simulink model "SistemaCAS_v9"  (R2014a)
settings: Solver=ode3  StartTime=0.0  StopTime=100  RelTol=1e-3
settings Model: Creator=andre  LastModifiedBy=andre

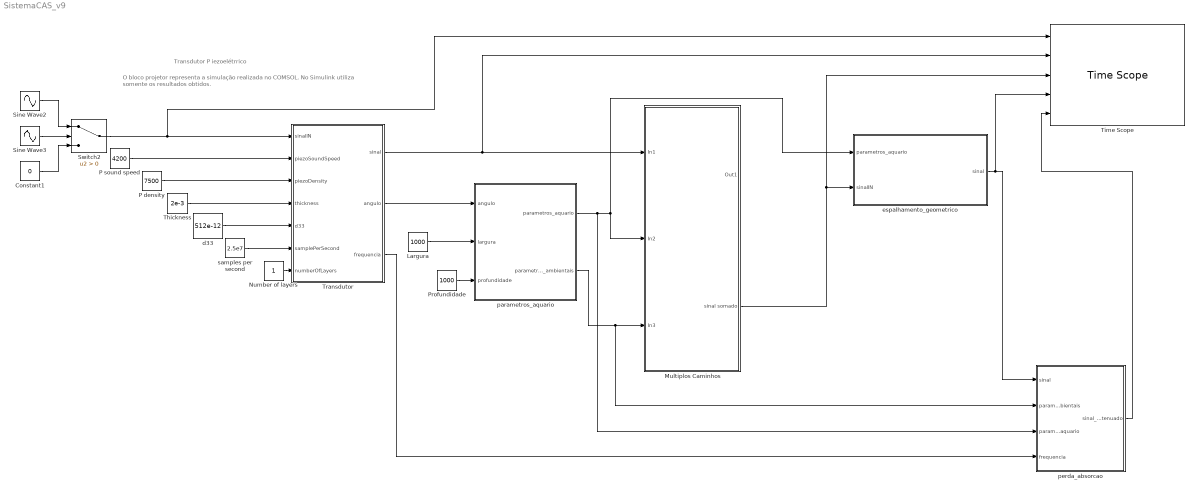
== system SistemaCAS_v9 ==
  note: O bloco projetor representa a simulação realizada no COMSOL. No Simulink utiliza somente os resultados obtidos.
  note: Transdutor P iezoelétrrico
  Constant1 : Constant  Value=0
  Largura : Constant  Value=1000
  Multiplos Caminhos : Subsystem
  Number of layers : Constant
  P density : Constant  Value=7500
  P sound speed : Constant  Value=4200
  Profundidade : Constant  Value=1000
  Sine Wave2 : Sin  SampleTime=0
  Sine Wave3 : Sin  SampleTime=0
  Switch2 : Switch  Criteria=u2 > Threshold
  Thickness : Constant  Value=2e-3
  Time Scope : TimeScope  NumInputPorts=5  DefaultConfigurationName=spbscopes.TimeScopeBlockCfg
  Transdutor : MATLAB Function  TreatAsAtomicUnit=on
  d33 : Constant  Value=512e-12
  espalhamento_geometrico : MATLAB Function  TreatAsAtomicUnit=on
  parametros_aquario : MATLAB Function  TreatAsAtomicUnit=on
  perda_absorcao : MATLAB Function  TreatAsAtomicUnit=on
  samples per second : Constant  Value=2.5e7
  wires:
  Largura/1 -> parametros_aquario/2(largura)
  Profundidade/1 -> parametros_aquario/3(profundidade)
  d33/1 -> Transdutor/5(d33)
  samples per second/1 -> Transdutor/6(samplePerSecond)
  Number of layers/1 -> Transdutor/7(numberOfLayers)
  P sound speed/1 -> Transdutor/2(piezoSoundSpeed)
  P density/1 -> Transdutor/3(piezoDensity)
  Thickness/1 -> Transdutor/4(thickness)
  Transdutor/2(angulo) -> parametros_aquario/1(angulo)
  Sine Wave2/1 -> Switch2/1
  Sine Wave3/1 -> Switch2/2
  Constant1/1 -> Switch2/3
  Switch2/1 -> Time Scope/1, Transdutor/1(sinalIN)
  Transdutor/1(sinal) -> Time Scope/2, Multiplos Caminhos/1(In1)
  parametros_aquario/1(parametros_aquario) -> perda_absorcao/3(parametros_aquario), Multiplos Caminhos/2(In2), espalhamento_geometrico/1(parametros_aquario)
  Multiplos Caminhos/2(sinal somado) -> Time Scope/3, espalhamento_geometrico/2(sinalIN)
  Transdutor/3(frequencia) -> perda_absorcao/4(frequencia)
  espalhamento_geometrico/1(sinal) -> Time Scope/4, perda_absorcao/1(sinal)
  parametros_aquario/2(parametros_ambientais) -> perda_absorcao/2(parametros_ambientais), Multiplos Caminhos/3(In3)
  perda_absorcao/1(sinal_atenuado) -> Time Scope/5

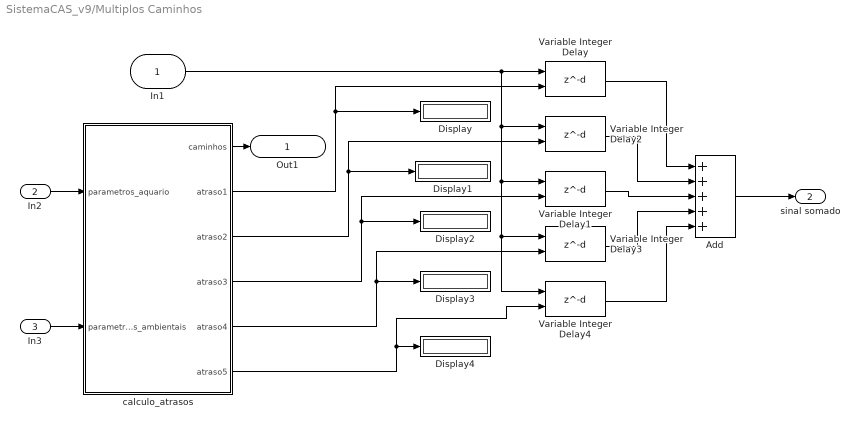
== system SistemaCAS_v9/Multiplos Caminhos ==
  In1 : Inport
  In2 : Inport  Port=2
  In3 : Inport  Port=3
  Add : Sum  Inputs=+++++
  Display{,1..4} (5 alike) : Display
  Variable Integer Delay{,1..4} (5 alike) : Delay  DelayLengthSource=Input port
      settings: InputPortMap=u0,p1
  calculo_atrasos : MATLAB Function  TreatAsAtomicUnit=on
  Out1 : Outport
  sinal somado : Outport  Port=2
  wires:
  calculo_atrasos/5(atraso4) -> Display3/1, Variable Integer Delay3/2
  calculo_atrasos/4(atraso3) -> Display2/1, Variable Integer Delay1/2
  In2/1 -> calculo_atrasos/1(parametros_aquario)
  In3/1 -> calculo_atrasos/2(parametros_ambientais)
  calculo_atrasos/1(caminhos) -> Out1/1
  In1/1 -> Variable Integer Delay4/1, Variable Integer Delay3/1, Variable Integer Delay1/1, Variable Integer Delay2/1, Variable Integer Delay/1
  calculo_atrasos/2(atraso1) -> Display/1, Variable Integer Delay/2
  calculo_atrasos/6(atraso5) -> Display4/1, Variable Integer Delay4/2
  Variable Integer Delay1/1 -> Add/3
  Variable Integer Delay2/1 -> Add/2
  Variable Integer Delay/1 -> Add/1
  Add/1 -> sinal somado/1
  calculo_atrasos/3(atraso2) -> Display1/1, Variable Integer Delay2/2
  Variable Integer Delay4/1 -> Add/5
  Variable Integer Delay3/1 -> Add/4

== matlab function SistemaCAS_v9/parametros_aquario ==
  data: angulo input; largura input; profundidade input; parametros_aquario output; parametros_ambientais output
function [parametros_aquario,parametros_ambientais] = parametros_aquario(angulo,largura,profundidade)
% consideraçoes para os parâmetros do aquário
% 1. emissor e receptor estão alinhados ( largura(x) e profundidade(z)
% iguais, só muda o comprimento (y)
% 2. o comprimento do aquario (L) é ideal para acontecer uma reflexão completa
% com o angulo de diretividade (que é o maior angulo possível do lóbulo 
% principal utilizando o transdutor piezoeletrico escolhido)
% 3. para facilitar os cálculos de do comprimento ideal, utilizamos largura
% igual profundidade (D = W)

% considerações sobre a simulação
% 1. serão considerados somente os caminhos do angulo de diretividade e o
% caminho direto (5 caminhos: um direto, dois que refletem nas laterais, e
% dois que refletem na superfície e o fundo
% 2. a reflexão será considerada reflexão completa com um eco (sem perdas 
% de energia ou refraçao)

%-------------------------------------------------------------------------
%Parâmetros do Aquário definidos anteriormente
%-------------------------------------------------------------------------
w = largura;                  % largura (eixo x)
d = profundidade;             % profundidade do aquário (eixo z) 
l = w/sin(angulo/2);      % comprimento do aquário calculado utilizando o angulo de diretividade (eixo y)
% l(éle) é a distancia ideal para acontecer uma reflexão completa
parametros_aquario = [w,l,d];


%-------------------------------------------------------------------------
% Valores dos parâmetros do meio subaquático 
%-------------------------------------------------------------------------
T = 30;                 % Temperatura (°C)
S = 1;                  % Salinidade (ppt)
pH = 7.2;               % acidêz da água - pH (potencial hidrogeniônico)
parametros_ambientais = [T, S, pH];

== matlab function SistemaCAS_v9/Multiplos Caminhos/calculo_atrasos ==
  data: caminhos output; atraso1 output; atraso2 output; atraso3 output; atraso4 output; atraso5 output; parametros_aquario input; parametros_ambientais input
function [caminhos,atraso1,atraso2,atraso3,atraso4,atraso5] = calculo_atrasos(parametros_aquario,parametros_ambientais)
%Definir as distâncias de cada caminho
%Atrasar o sinal de cada caminho
%Enviar a distância e o sinal de cada caminho ()

w = parametros_aquario(1);
l = parametros_aquario(2);
d = parametros_aquario(3);

T = parametros_ambientais(1);
S = parametros_ambientais(2);
pH = parametros_ambientais(3);

%%%%%%  Bloco multipath  %%%%%%

%-------------------------------------------------------------------------
%Definindo as distâncias de cada caminho do multipath
%-------------------------------------------------------------------------
% caminho_1 = caminho refletido na superfície
% caminho_2 = caminho refletido na lateral de trás
% caminho_3 = caminho direto
% caminho_4 = caminho refletido na lateral da frente
% caminho_5 = caminho refletido no fundo
caminhos = [0 0 0 0 0];
caminhos(1) = sqrt(d^2 + l^2);
caminhos(2) = sqrt(w^2 + l^2);
caminhos(3) = l;
caminhos(4) = caminhos(2);
caminhos(5) = caminhos(1);

%-------------------------------------------------------------------------
%Definindo a profundidade média para cada caminho
%-------------------------------------------------------------------------
D = [0 0 0 0 0];
D(1) = mean([d/2,0]);
D(2) = d/2;
D(3) = d/2;
D(4) = d/2;
D(5) = mean([d,d/2]);

%-------------------------------------------------------------------------
%Velocidade do som na água (m/s)
%-------------------------------------------------------------------------
C = [0 0 0 0 0];
for i = 1:5 %5 caminhos
    c = 1448.96 + 4.591*T - 5.304*(10^(-2))*(T^(2))...
        + 2.374*(10^(-4))*(T^(3)) + 1.340*(S-35) + 1.630*(10^(-2))*D(i)...
        + 1.675*(10^(-7))*(D(i)^(2)) - 1.025*(10^(-2))*T*(S-35)...
        - 7.139*(10^(-13))*T*(D(i)^(3));
    
    %Conversão de (m/s) para (cm/s)
    C(i)=c*100;
end

%-------------------------------------------------------------------------
% Definindo os atrasos de cada caminho do multipath através da equação de
% velocidade de propagação do som na água
%-------------------------------------------------------------------------

% atraso é o tempo que o caminho leva

atraso1 = 100*D(1)/C(1);
atraso2 = 100*D(2)/C(2);
atraso3 = 100*D(3)/C(3); % caminho direto não tem atraso
atraso4 = 100*D(4)/C(4);
atraso5 = 100*D(5)/C(5);

== matlab function SistemaCAS_v9/perda_absorcao ==
  data: sinal input; parametros_ambientais input; parametros_aquario input; frequencia input; sinal_atenuado output
function sinal_atenuado = perda_absorcao(sinal,parametros_ambientais,parametros_aquario,frequencia)

% Parâmetros Ambientais
T = parametros_ambientais(1);
S = parametros_ambientais(2);
pH = parametros_ambientais(3);

%Profundidade
D = parametros_aquario(3);

%Valores dos parâmetros Ácido Bórico(f1) e Sulfato de Magnésio(f2)
f1 = 0.78 * sqrt(S/35) * (exp(T/26));
f2 = 42 * (exp(T/17));

%Absorption Coefficient
a = ((0.106 * (f1 * frequencia^2) * exp((pH - 8)/0.56)) / (f1^2 + frequencia^2)) +...
    ((0.52 * (1 + (T/43)) * (S/45) * (f2 * frequencia^2) *...
    exp(-(D/6))) / (f2^2 + frequencia^2)) + (0.00049 * (frequencia^2) * (exp(-(T/27 + D/17))));

sinal_atenuado = sinal + a;

== matlab function SistemaCAS_v9/espalhamento_geometrico ==
  data: parametros_aquario input; sinal output; sinalIN input
function sinal = espalhamento_geometrico(parametros_aquario,sinalIN)

% ONDE ESTÁ O FATOR K?????


%utilizano espalhamento geométrico cilíndrico 
% utilizar cálculos abaixo
%(https://dosits.org/science/advanced-topics/cylindrical-vs-spherical-spreading/)

r = parametros_aquario(2); % referente à largura do aquário
%perda_espalhamento =  10*log10(r);

sinal = sinalIN/r;

== matlab function SistemaCAS_v9/Transdutor ==
  data: sinalIN input; sinal output; piezoSoundSpeed input; piezoDensity input; thickness input; d33 input; samplePerSecond input; numberOfLayers input; angulo output; frequencia output
function [sinal, angulo, frequencia] = projetor(sinalIN, piezoSoundSpeed, piezoDensity, thickness, d33, samplePerSecond, numberOfLayers)


%-------------------------------------------------------------------------
% Sinal 
%-------------------------------------------------------------------------
sinal=sinalIN;

%-------------------------------------------------------------------------
% Ângulo de diretividade do transdutor calculado no COMSOL (rad)
%-------------------------------------------------------------------------
angulo = pi/3;            % (ex.: 60º = pi/3 rad)

%-------------------------------------------------------------------------
% Frequência do Sinal (kHz)
%-------------------------------------------------------------------------
frequencia = 1000;
